simulink model "Simple_Model_v2"  (R2023a)
settings: Solver=VariableStepAuto  StartTime=0.0  StopTime=1000  RelTol=1e-3
libraries: dspsigops x1
settings Model: Creator=levir  LastModifiedBy=levir

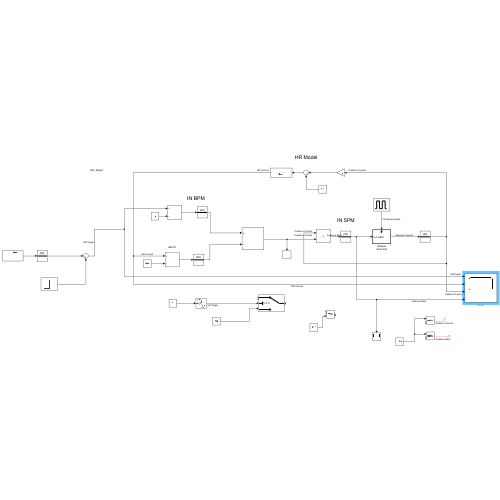
[thumbnail: Simulink's stored preview of the top-level diagram]
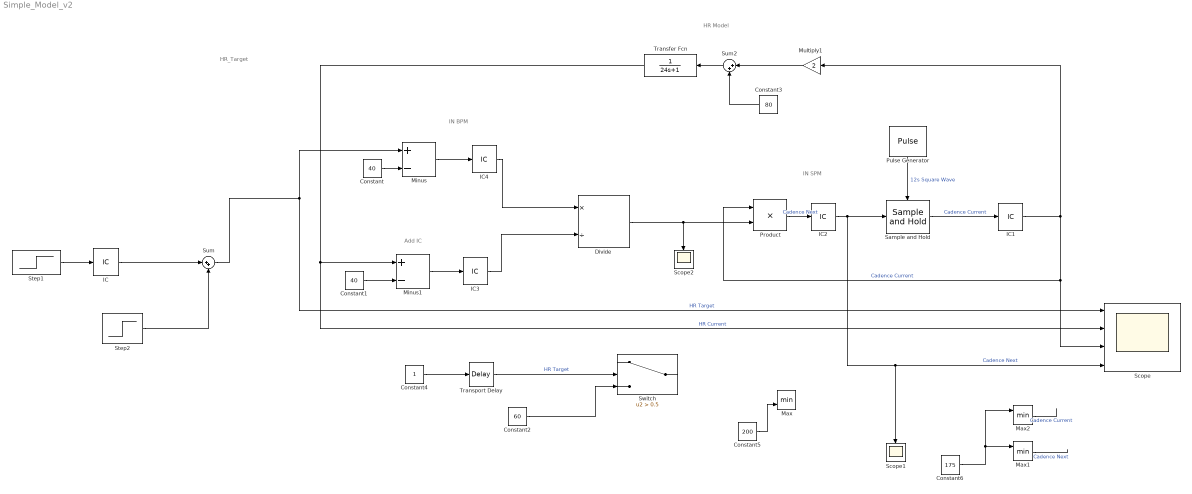
== system Simple_Model_v2 ==
  note: HR Model
  note: IN BPM
  note: IN SPM
  note: HR_Target
  note: Add IC
  Constant : Constant  Value=40
  Constant1 : Constant  Value=40
  Constant2 : Constant  Value=60
  Constant3 : Constant  Value=80
  Constant4 : Constant
  Constant5 : Constant  Value=200
  Constant6 : Constant  Value=175
  Divide : Product  Inputs=*/
  IC{,1..4} (5 alike) : InitialCondition  Value=60
  Max : MinMax  Inputs=2
  Max1 : MinMax  Inputs=2
  Max2 : MinMax  Inputs=2
  Minus : Sum  Inputs=+-
  Minus1 : Sum  Inputs=+-
  Multiply1 : Gain  Gain=2
  Product : Product
  Pulse Generator : DiscretePulseGenerator  PulseType=Time based  Period=10  PulseWidth=10
  Sample and Hold : dspsigops/Sample and Hold  trig=Rising edge  initCond=150  latchinput=on
  Scope : Scope  NumInputPorts=4
  Scope1 : Scope
  Scope2 : Scope
  Step1 : Step  After=130  SampleTime=0
  Step2 : Step  Time=350  After=50  SampleTime=0
  Sum : Sum  Inputs=|++
  Sum2 : Sum  Inputs=|++
  Switch : Switch  Criteria=u2 > Threshold  Threshold=0.5  SaturateOnIntegerOverflow=off  InputSameDT=off
  Transfer Fcn : TransferFcn  Denominator=[24 1]
  Transport Delay : TransportDelay  DelayTime=15
  wires:
  Sum2/1 -> Transfer Fcn/1
  Sum/1 -> Minus/1, Scope/1  "HR Target"
  Multiply1/1 -> Sum2/1
  Sample and Hold/1 -> IC1/1  "Cadence Current"
  Constant3/1 -> Sum2/2
  Product/1 -> IC2/1  "Cadence Next"
  Constant1/1 -> Minus1/2
  Constant/1 -> Minus/2
  Minus1/1 -> IC3/1
  Pulse Generator/1 -> Sample and Hold/Trigger  "12s Square Wave"
  Minus/1 -> IC4/1
  Divide/1 -> Product/2, Scope2/1
  Transport Delay/1 -> Switch/2  "HR Target"
  Constant2/1 -> Switch/3
  Transfer Fcn/1 -> Scope/2, Minus1/1  "HR Current"
  Constant4/1 -> Transport Delay/1
  Step1/1 -> IC/1
  Step2/1 -> Sum/2
  IC/1 -> Sum/1
  IC1/1 -> Multiply1/1, Product/1, Scope/3  "Cadence Current"
  IC2/1 -> Scope1/1, Scope/4, Sample and Hold/1  "Cadence Next"
  IC3/1 -> Divide/2
  IC4/1 -> Divide/1
  Constant5/1 -> Max/2
  Max1/1 -> ?  "Cadence Next"
  Constant6/1 -> Max2/1, Max1/1
  Max2/1 -> ?  "Cadence Current"
